simulink model "BLOCKrigged"  (Simulink 7.9)
settings: Solver=ode45  StartTime=0.0  StopTime=6  RelTol=1e-3
settings Model: Creator=Nick  LastModifiedBy=Nick

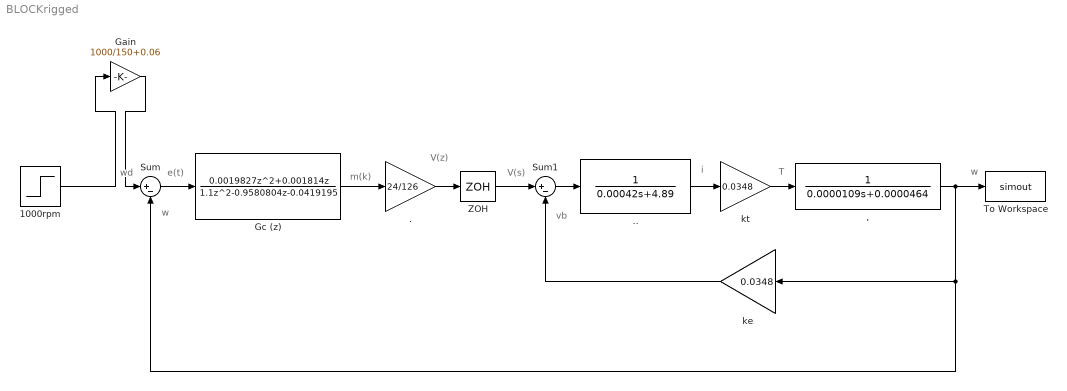
== system BLOCKrigged ==
  note: wd
  note: e(t)
  note: m(k)
  note: V(z)
  note: V(s)
  note: vb
  note: w
  note: i
  note: T
  note: w
  , : TransferFcn  Denominator=[0.0000109 0.0000464]
  . : Gain  Gain=24/126  SampleTime=0.004
  .. : TransferFcn  Denominator=[0.00042 4.89]
  1000rpm : Step  Time=0  After=2000  SampleTime=0.004
  Gain : Gain  Gain=1000/150+0.06
  Gc (z) : DiscreteTransferFcn  Tag=z  Numerator=[0.0019827 0.001814 0]  Denominator=[1.1 -0.9580804 -0.0419195]  SampleTime=0.004
  Sum : Sum  Inputs=|+-  SampleTime=0.004
  Sum1 : Sum  Inputs=|+-  SampleTime=0.004
  To Workspace : ToWorkspace  VariableName=simout  SampleTime=0.004
  ZOH : ZeroOrderHold  SampleTime=0.004
  ke : Gain  Gain=0.0348  SampleTime=0.004
  kt : Gain  Gain=0.0348  SampleTime=0.004
  wires:
  Sum/1 -> Gc (z)/1
  Gc (z)/1 -> ./1
  ./1 -> ZOH/1
  ZOH/1 -> Sum1/1
  ke/1 -> Sum1/2
  1000rpm/1 -> Gain/1
  Sum1/1 -> ../1
  ../1 -> kt/1
  kt/1 -> ,/1
  ,/1 -> Sum/2, ke/1, To Workspace/1
  Gain/1 -> Sum/1
